simulink model "control_colas"  (R2023a)
settings: Solver=VariableStepAuto  StartTime=0.0  StopTime=25  RelTol=1e-3
undefined symbols (not defined in the file or in its folder): m
settings Model: Creator=santi  LastModifiedBy=santi

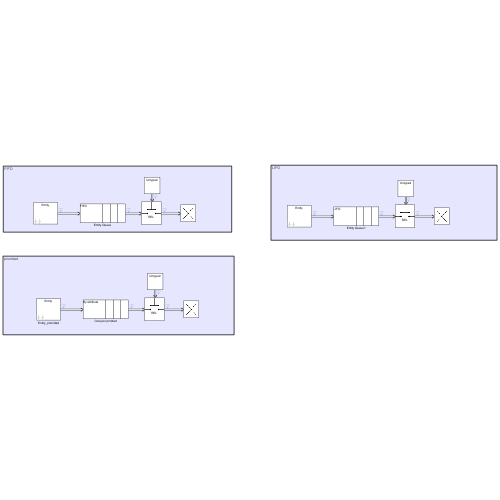
[thumbnail: Simulink's stored preview of the top-level diagram]
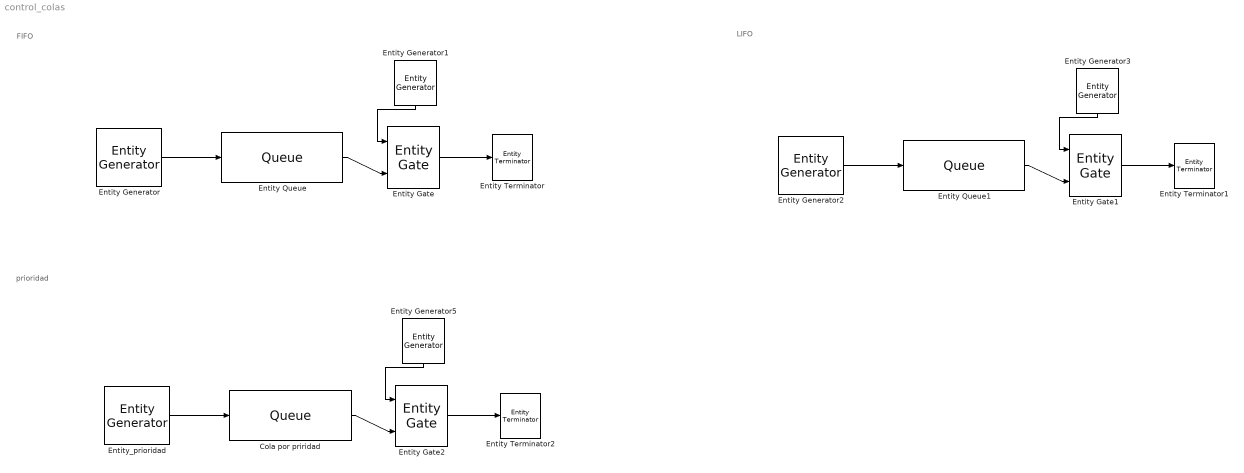
== system control_colas ==
  note: prioridad
  note: LIFO
  note: FIFO
  Cola por priridad : Queue  InputPortMessageModes=m  OutputPortMessageModes=m  QueueType=Priority  PrioritySource=attribute  SortingDirection=Descending
  Entity Gate : EntityGate  InputPortMessageModes=m,m  OutputPortMessageModes=m  OperatingMode=Release gate
  Entity Gate1 : EntityGate  InputPortMessageModes=m,m  OutputPortMessageModes=m  OperatingMode=Release gate
  Entity Gate2 : EntityGate  InputPortMessageModes=m,m  OutputPortMessageModes=m  OperatingMode=Release gate
  Entity Generator : EntityGenerator  OutputPortMessageModes=m  TimeSource=MATLAB action  IntergenerationTimeAction=|  GenerateEntityAtSimulationStart=off  GenerateAction=|  AttributeName=attribute  EntityType=Structured  EntityTypeName=Entity
      IntergenerationTimeAction=|
      | % Patrón de repetición de secuencia
      | % Se inicializan las variables
      | persistent SEC;
      | persistent idx;
      | if isempty(SEC)
      |     % Se generan 10 entidades con 1 segundo de intervalo
      |     SEC = [1 1 1 1 1 1 1 1 1 1];
      |     idx = 1;
      | end
      | if idx > numel(SEC)
      |     % Se detiene la generación de entidades después de 10
      |     dt = inf;
      |     else
      |         dt = SEC(idx);
      | end
      | idx = idx + 1;
      GenerateAction=|
      | % Se modifica el valor del atributo de la entidad en cada paso de reloj.
      | persistent SEC1;
      | persistent idx1;
      | if isempty(SEC1)
      |     SEC1 = [1 2 3 4 5 6 7 8 9 10];
      |     idx1 = 1;
      | end
      | if idx1 <= numel(SEC1)
      |     entity.attribute = SEC1(idx1);
      | end
      | idx1 = idx1 + 1;
  Entity Generator1 : EntityGenerator  OutputPortMessageModes=m  TimeSource=MATLAB action  IntergenerationTimeAction=|  GenerateEntityAtSimulationStart=off  AttributeName=entity  AttributeInitialValue=0  EntityTypeName=Entity
      | % Cada valor de la secuencia representa el retardo en liberar las entidades
      | % de la cola
      | persistent SEC;
      | persistent idx;
      | if isempty(SEC)
      |     SEC = [10 1 1 1 1 1 1 1 1 1];
      |     idx = 1;
      | end
      | if idx > numel(SEC)
      |     dt= inf;
      |     else
      |         dt = SEC(idx);
      | end
      | idx = idx + 1;
  Entity Generator2 : EntityGenerator  OutputPortMessageModes=m  TimeSource=MATLAB action  IntergenerationTimeAction=|  GenerateEntityAtSimulationStart=off  GenerateAction=|  AttributeName=attribute  EntityType=Structured  EntityTypeName=Entity
      IntergenerationTimeAction=|
      | % Patrón de repetición de secuencia
      | % Se inicializan las variables
      | persistent SEC;
      | persistent idx;
      | if isempty(SEC)
      |     % Se generan 10 entidades con 1 segundo de intervalo
      |     SEC = [1 1 1 1 1 1 1 1 1 1];
      |     idx = 1;
      | end
      | if idx > numel(SEC)
      |     % Se detiene la generación de entidades después de 10
      |     dt = inf;
      |     else
      |         dt = SEC(idx);
      | end
      | idx = idx + 1;
      GenerateAction=|
      | % Se modifica el valor del atributo de la entidad en cada paso de reloj.
      | persistent SEC1;
      | persistent idx1;
      | if isempty(SEC1)
      |     SEC1 = [1 2 3 4 5 6 7 8 9 10];
      |     idx1 = 1;
      | end
      | if idx1 <= numel(SEC1)
      |     entity.attribute = SEC1(idx1);
      | end
      | idx1 = idx1 + 1;
  Entity Generator3 : EntityGenerator  OutputPortMessageModes=m  TimeSource=MATLAB action  IntergenerationTimeAction=|  GenerateEntityAtSimulationStart=off  AttributeName=entity  AttributeInitialValue=0  EntityTypeName=Entity
      | % Cada valor de la secuencia representa el retardo en liberar las entidades
      | % de la cola
      | persistent SEC;
      | persistent idx;
      | if isempty(SEC)
      |     SEC = [11 1 1 1 1 1 1 1 1 1];
      |     idx = 1;
      | end
      | if idx > numel(SEC)
      |     dt= inf;
      |     else
      |         dt = SEC(idx);
      | end
      | idx = idx + 1;
  Entity Generator5 : EntityGenerator  OutputPortMessageModes=m  TimeSource=MATLAB action  IntergenerationTimeAction=|  GenerateEntityAtSimulationStart=off  AttributeName=entity  AttributeInitialValue=0  EntityTypeName=Entity
      | % Cada valor de la secuencia representa el retardo en liberar las entidades
      | % de la cola
      | persistent SEC;
      | persistent idx;
      | if isempty(SEC)
      |     SEC = [10 1 1 1 1 1 1 1 1 1];
      |     idx = 1;
      | end
      | if idx > numel(SEC)
      |     dt= inf;
      |     else
      |         dt = SEC(idx);
      | end
      | idx = idx + 1;
  Entity Queue : Queue  InputPortMessageModes=m  OutputPortMessageModes=m
  Entity Queue1 : Queue  InputPortMessageModes=m  OutputPortMessageModes=m  QueueType=LIFO
  Entity Terminator : EntityTerminator  InputPortMessageModes=m
  Entity Terminator1 : EntityTerminator  InputPortMessageModes=m
  Entity Terminator2 : EntityTerminator  InputPortMessageModes=m
  Entity_prioridad : EntityGenerator  OutputPortMessageModes=m  TimeSource=MATLAB action  IntergenerationTimeAction=|  GenerateEntityAtSimulationStart=off  GenerateAction=|  AttributeName=attribute  EntityType=Structured  EntityTypeName=Entity
      IntergenerationTimeAction=|
      | % Patrón de repetición de secuencia
      | % Se inicializan las variables
      | persistent SEC;
      | persistent idx;
      | if isempty(SEC)
      |     % Se generan 10 entidades con 1 segundo de intervalo
      |     SEC = [1 1 1 1 1 1 1 1 1 1];
      |     idx = 1;
      | end
      | if idx > numel(SEC)
      |     % Se detiene la generación de entidades después de 10
      |     dt = inf;
      |     else
      |         dt = SEC(idx);
      | end
      | idx = idx + 1;
      GenerateAction=|
      | % Se modifica el valor del atributo de la entidad en cada paso de reloj.
      | persistent SEC1;
      | persistent idx1;
      | if isempty(SEC1)
      |     SEC1 = [1 2 3 4 5 6 7 8 9 10];
      |     idx1 = 1;
      | end
      | if idx1 <= numel(SEC1)
      |     entity.attribute = SEC1(idx1);
      | end
      | idx1 = idx1 + 1;
  wires:
  Entity Generator/1 -> Entity Queue/1
  Entity Queue/1 -> Entity Gate/2
  Entity Gate/1 -> Entity Terminator/1
  Entity Generator1/1 -> Entity Gate/1
  Entity Queue1/1 -> Entity Gate1/2
  Entity Gate1/1 -> Entity Terminator1/1
  Entity Generator3/1 -> Entity Gate1/1
  Entity Generator2/1 -> Entity Queue1/1
  Cola por priridad/1 -> Entity Gate2/2
  Entity Gate2/1 -> Entity Terminator2/1
  Entity Generator5/1 -> Entity Gate2/1
  Entity_prioridad/1 -> Cola por priridad/1
